simulink model "rednoise_corr_signal_v1"  (R2022b)
settings: Solver=VariableStepAuto  StartTime=0.0  StopTime=1000  RelTol=1e-3
libraries: simulink x1, dspsrcs4 x1
settings Model: Creator=shukl  LastModifiedBy=shukl

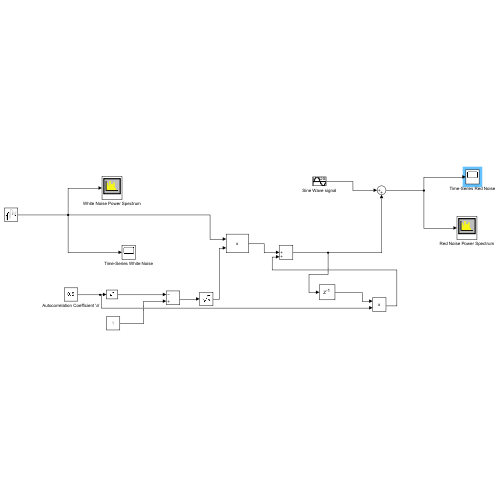
[thumbnail: Simulink's stored preview of the top-level diagram]
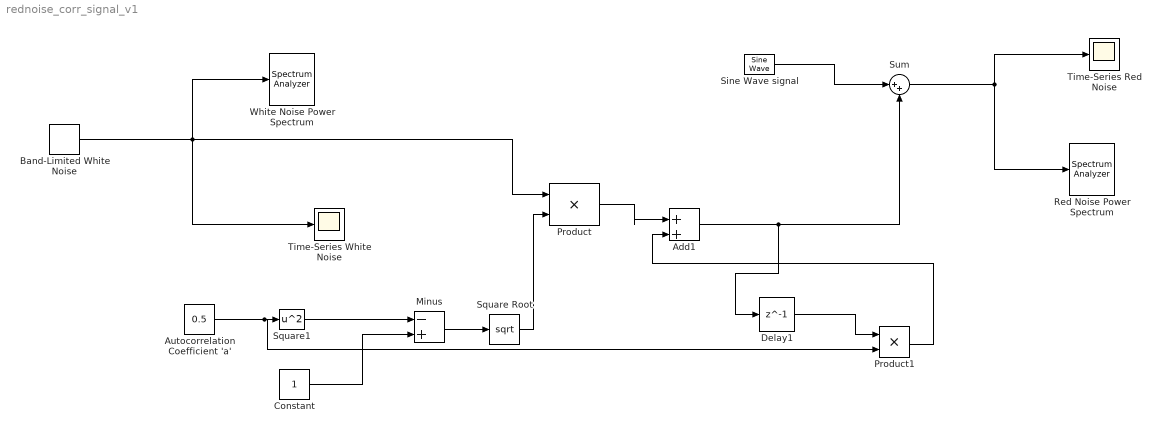
== system rednoise_corr_signal_v1 ==
  Add1 : Sum  Inputs=|++
  Autocorrelation Coefficient 'a' : Constant  Value=0.5
  Band-Limited White Noise : simulink/Sources/Band-Limited White Noise  Cov=[0.1]  Ts=0.1  seed=[23341]
  Constant : Constant
  Delay1 : Delay  DelayLength=1
  Minus : Sum  Inputs=-+
  Product : Product
  Product1 : Product
  Red Noise Power Spectrum : SpectrumAnalyzer
  Sine Wave signal : dspsrcs4/Sine Wave  Amplitude=1  Frequency=3  Phase=0  SampleMode=Discrete  OutComplex=Real  CompMethod=Trigonometric fcn  TableSize=Speed  SampleTime=0.1  SamplesPerFrame=1  ResetState=Restart at time zero  OutputFrames=off  dataType=double  wordLen=16  udDataType=sfix(16)  fracBitsMode=Best precision  numFracBits=15  OutDataTypeStr=double  LastOutDataTypeStr=double
  Square Root : Sqrt
  Square1 : Math  Operator=square
  Sum : Sum  Inputs=|++
  Time-Series Red Noise : Scope
  Time-Series White Noise : Scope
  White Noise Power Spectrum : SpectrumAnalyzer
  wires:
  Band-Limited White Noise/1 -> Time-Series White Noise/1, Product/1, White Noise Power Spectrum/1
  Add1/1 -> Sum/2, Delay1/1
  Delay1/1 -> Product1/1
  Product1/1 -> Add1/2
  Product/1 -> Add1/1
  Sine Wave signal/1 -> Sum/1
  Sum/1 -> Time-Series Red Noise/1, Red Noise Power Spectrum/1
  Square1/1 -> Minus/1
  Minus/1 -> Square Root/1
  Square Root/1 -> Product/2
  Constant/1 -> Minus/2
  Autocorrelation Coefficient 'a'/1 -> Square1/1, Product1/2
